simulink model "Fouromniwheel"  (R2020a)
settings: Solver=VariableStepAuto  StartTime=0.0  StopTime=inf  RelTol=1e-3  EnableMultiTasking=on
libraries: mobileRoboticsLib x4
settings Model: Creator=ADMIN  LastModifiedBy=RAJENDRA PHUTANE
settings DataIOCC: LimitDataPoints=on  MaxDataPoints=10000
settings OptimizationCC: LifeSpan=inf
settings DebuggingCC: AllowSymbolicDim=off  SFUnexpectedBacktrackingDiag=warning  SFNoUnconditionalDefaultTransitionDiag=warning  SFExecutionAtInitializationDiag=none  ArithmeticOperatorsInVariantConditions=warning
settings SFSimCC: SimUseLocalCustomCode=off  CustomCodeUndefinedFunction=UseInterfaceOnly
settings RTWCC: RTWUseLocalCustomCode=off
settings CodeAppCC: StateflowObjectComments=on
settings GRTTargetCC: TargetLangStandard=C89/C90 (ANSI)
settings ConfigComp: CovMetricSettings=dw  CovHtmlReporting=on  CovSaveCumulativeToWorkspaceVar=on  CovSaveSingleToWorkspaceVar=on  CovExternalEMLEnable=off  CovSFcnEnable=off
settings SimscapeCC: SimscapeLogType=all  SimscapeLogSimulationStatistics=on  SimscapeLogDataHistory=10000

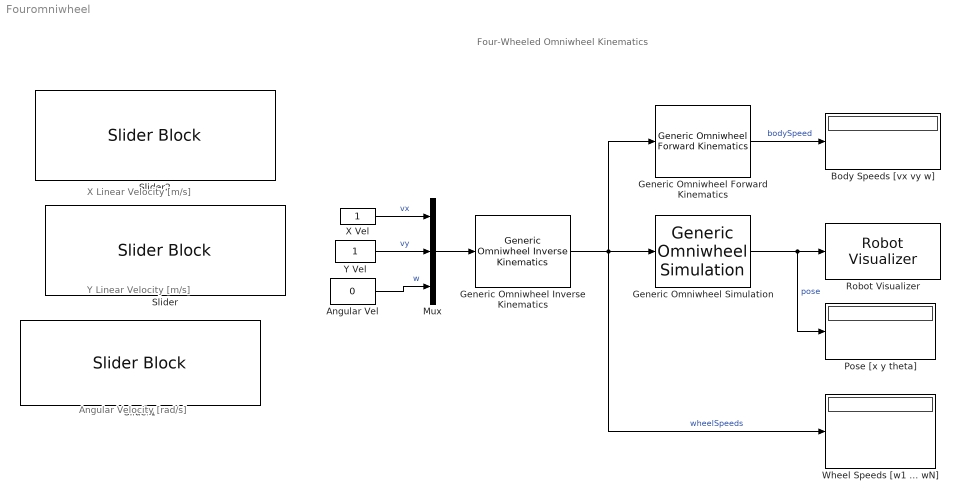
== system Fouromniwheel ==
  note: X Linear Velocity [m/s]
  note: Y Linear Velocity [m/s]
  note: Angular Velocity [rad/s]
  note: Four-Wheeled Omniwheel Kinematics
  Angular Vel : Constant  Value=0
  Body Speeds [vx vy w] : Display
  Generic Omniwheel Forward Kinematics : mobileRoboticsLib/Kinematic Models/Generic Omniwheel/Generic Omniwheel  Forward Kinematics  wheelRadius=PR.wheelRadius  wheelPositions=PR.wheelPositions  wheelAngles=PR.wheelAngles
      settings: SourceProductName=Mobile Robotics Simulation Toolbox
  "Generic Omniwheel Inverse Kinematics " : mobileRoboticsLib/Kinematic Models/Generic Omniwheel/Generic Omniwheel  Inverse Kinematics   wheelRadius=PR.wheelRadius  wheelPositions=PR.wheelPositions  wheelAngles=PR.wheelAngles
      settings: SourceProductName=Mobile Robotics Simulation Toolbox
  Generic Omniwheel Simulation : mobileRoboticsLib/Kinematic Models/Generic Omniwheel/Generic Omniwheel Simulation  wheelRadius=PR.wheelRadius  wheelPositions=PR.wheelPositions  wheelAngles=PR.wheelAngles  initX=0  initY=0  initAngle=0  Ts=0.05
      settings: SourceProductName=Mobile Robotics Simulation Toolbox
  Mux : Mux  Inputs=3
  Pose [x y theta] : Display
  Robot Visualizer : mobileRoboticsLib/Environments/Robot Visualizer  Priority=99  robotRadius=PR.RobotRadius  showTrajectory=on  hasWaypoints=off  hasLidar=off  sensorOffset=[ 0 0 ]  scanAngles=scanAngles  hasObjDetector=off  objDetectorOffset=[ 0, 0 ]  objDetectorAngle=0  objDetectorFOV=pi/4  objDetectorMaxRange=5  objectColors=[ 1, 0, 0; 0, 1, 0; 0, 0, 1 ]  objectMarkers=s
  Slider : SliderBlock  ScaleMin=-1  ScaleMax=1  TickInterval=0.25
  Slider1 : SliderBlock  ScaleMin=-1.5  ScaleMax=1.5  TickInterval=0.5
  Slider2 : SliderBlock  ScaleMin=-1  ScaleMax=1  TickInterval=0.25
  Wheel Speeds [w1 ... wN] : Display
  X Vel : Constant
  Y Vel : Constant
  wires:
  Angular Vel/1 -> Mux/3  "w"
  "Generic Omniwheel Inverse Kinematics "/1 -> Generic Omniwheel Simulation/1, Generic Omniwheel Forward Kinematics/1, Wheel Speeds [w1 ... wN]/1  "wheelSpeeds"
  X Vel/1 -> Mux/1  "vx"
  Generic Omniwheel Simulation/1 -> Pose [x y theta]/1, Robot Visualizer/1  "pose"
  Y Vel/1 -> Mux/2  "vy"
  Mux/1 -> "Generic Omniwheel Inverse Kinematics "/1
  Generic Omniwheel Forward Kinematics/1 -> Body Speeds [vx vy w]/1  "bodySpeed"
